simulink model "base_model_1_"  (R2025b)
settings: Solver=FixedStepAuto  StartTime=0.0  StopTime=864000  FixedStep=3600  RelTol=1e-3
undefined symbols (not defined in the file or in its folder): DiscIntNeverNeededParam
settings Model: SimulationMode=accelerator  Creator=Gmusl  LastModifiedBy=caddo

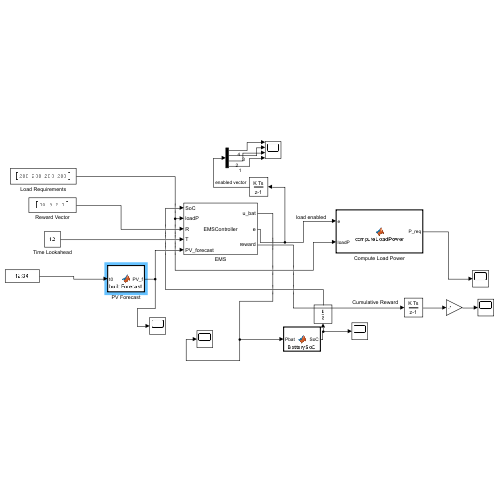
[thumbnail: Simulink's stored preview of the top-level diagram]
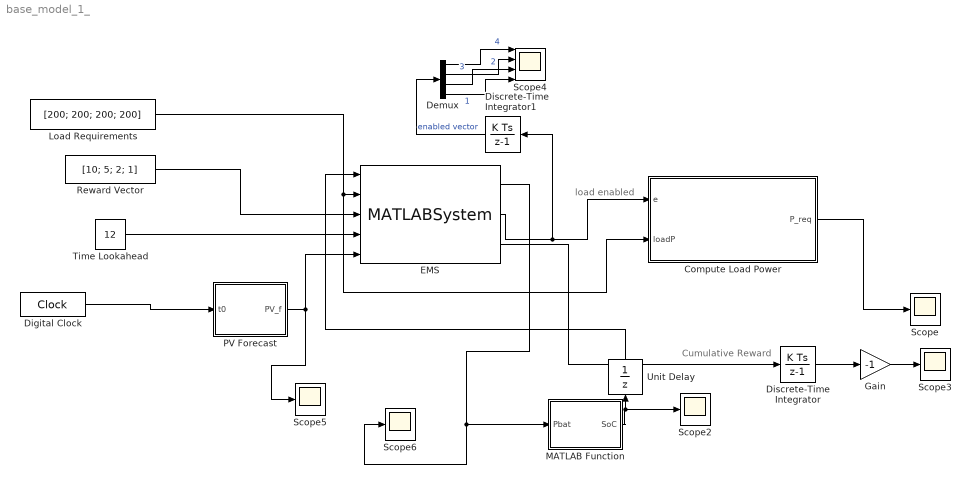
== system base_model_1_ ==
  note: Cumulative Reward
  note: load enabled
  Compute Load Power : MATLAB Function  TreatAsAtomicUnit=on
  Demux : Demux
  Digital Clock : DigitalClock  SampleTime=3600
  Discrete-Time Integrator : DiscreteIntegrator  SampleTime=-1  ICPrevOutput=DiscIntNeverNeededParam  ICPrevScaledInput=DiscIntNeverNeededParam
  Discrete-Time Integrator1 : DiscreteIntegrator  SampleTime=-1  ICPrevOutput=DiscIntNeverNeededParam  ICPrevScaledInput=DiscIntNeverNeededParam
  EMS : MATLABSystem  System=EMSController  SimulateUsing=Interpreted execution
      mask Type: EMSController
  Gain : Gain  Gain=-1
  Load Requirements : Constant  Value=[200; 200; 200; 200]
  MATLAB Function : MATLAB Function  TreatAsAtomicUnit=on
  PV Forecast : MATLAB Function  TreatAsAtomicUnit=on
  Reward Vector : Constant  Value=[10; 5; 2; 1]
  Scope{,2..3,5..6} (5 alike) : Scope
      Scope settings: ActiveDisplayYMinimum=-923.10828007434134  ActiveDisplayYMaximum=4981.0470479433025
      Scope2 settings: ActiveDisplayYMinimum=0.10625000000000004  ActiveDisplayYMaximum=1.04375  DataLoggingVariableName=ScopeData2
      Scope3 settings: ActiveDisplayYMinimum=-9.29846668459104E+6  ActiveDisplayYMaximum=1.1472480368843886E+8  DataLoggingVariableName=ScopeData3
      Scope5 settings: ActiveDisplayYMinimum=-267.19305037896061  ActiveDisplayYMaximum=1013.2291963980758  DataLoggingVariableName=ScopeData5
      Scope6 settings: ActiveDisplayYMinimum=-1191.1457713116706  ActiveDisplayYMaximum=1458.6422273256735  DataLoggingVariableName=ScopeData6
  Scope4 : Scope  NumInputPorts=4
      settings: ActiveDisplayYMinimum=-97254.198849255219  ActiveDisplayYMaximum=492349.35112402204  DataLoggingVariableName=ScopeData4
  Time Lookahead : Constant  Value=12
  Unit Delay : UnitDelay  SampleTime=-1  HasFrameUpgradeWarning=on
  wires:
  MATLAB Function/1(SoC) -> Unit Delay/1, Scope2/1
  Time Lookahead/1 -> EMS/4
  Load Requirements/1 -> Compute Load Power/2(loadP), EMS/2
  Reward Vector/1 -> EMS/3
  EMS/2 -> Discrete-Time Integrator1/1, Compute Load Power/1(e)
  Compute Load Power/1(P_req) -> Scope/1
  Digital Clock/1 -> PV Forecast/1(t0)
  PV Forecast/1(PV_f) -> EMS/5, Scope5/1
  Demux/1 -> Scope4/1  "4"
  Demux/2 -> Scope4/2  "3"
  Demux/3 -> Scope4/3  "2"
  Demux/4 -> Scope4/4  "1"
  EMS/3 -> Discrete-Time Integrator/1
  Discrete-Time Integrator/1 -> Gain/1
  Gain/1 -> Scope3/1
  EMS/1 -> MATLAB Function/1(Pbat), Scope6/1
  Discrete-Time Integrator1/1 -> Demux/1  "enabled vector"
  Unit Delay/1 -> EMS/1

== matlab function base_model_1_/PV Forecast ==
  data: t0 input size=[1 1]; PV_f output size=[12 1]
function PV_f = buildForecast(t0)
%#codegen

dt = 3600;             % 1 hour per step
Pmax = 1200;           
day_length = 86400;   

T = 12;

PV_f = zeros(T,1);  % fixed-size

for k = 1:T
    t_future = t0 + k*dt;
    PV_f(k) = max(Pmax * sin(pi * t_future / day_length), 0);
end
end

== matlab function base_model_1_/MATLAB Function ==
  data: Pbat input; SoC output
function SoC = BatterySoC(Pbat)
% Pbat is the battery power command in Watts

persistent soc_state

% Parameters
Ts = 1;       % sample time (sec)
E_nom = 10000;   % battery energy capacity (Wh)
eta_c = 0.98;
eta_d = 0.98;

% Initialize persistent SoC if empty
if isempty(soc_state)
    soc_state = 0.5;   % initial SoC (50%)
end

% Separate into charge and discharge
P_ch  = max(Pbat, 0);     % charging power
P_dis = max(-Pbat, 0);    % discharging power

% ΔSoC update
dSoC = (Ts/E_nom) * (eta_c * P_ch - (1/eta_d) * P_dis);

% Update
soc_state = soc_state + dSoC;

% Limit SoC between 0.2 and 0.9
soc_state = min(max(soc_state, 0.2), 0.9);

% Output
SoC = soc_state;

== matlab function base_model_1_/Compute Load Power ==
  data: e input; P_req output; loadP input
function P_req = computeLoadPower(e, loadP)
% e      : vector of enable signals (0/1)
% loadP  : vector of load power ratings (W)
% Output : total required load power (W)

    % Ensure column vectors
    e = e(:);
    loadP = loadP(:);

    % Total load power
    P_req = sum(e .* loadP);
end
